simulink model "BLDC_Completo"  (R2024b)
settings: Solver=ode23s  StartTime=0.0  StopTime=3  MaxStep=1e-4  RelTol=1e-3
values from neighbouring files (symbols this model uses):
  b_eq = b_l*(1/r)^2+b_m    (= 2.36823386114e-05)    [Parametros.m]
  c_pitch = cos(pitch)    [Parametros.m]
  J_eq = J_l*(1/r)^2+J_m    (= 7.12145792242e-06)    [Parametros.m]
  K_e = 0.0217    [Parametros.m]
  k_l = m*g*l_cm+m_l*g*l_l    (= 5.05042475)    [Parametros.m]
  K_t = 21.7e-3    (= 0.0217)    [Parametros.m]
  Kd_m = J_eq*n*w_pos    (= 0.0159520657462)    [Parametros.m]
  ke_int = w_obs^3    (= 125000000000)    [Parametros.m]
  ke_tita = w_obs*3    (= 15000)    [Parametros.m]
  ke_w = 3*w_obs^2    (= 75000000)    [Parametros.m]
  Ki_m = J_eq*w_pos^3    (= 3646.18645628)    [Parametros.m]
  Kp_m = J_eq*n*w_pos^2    (= 12.761652597)    [Parametros.m]
  L_s = 0.113e-3    (= 0.000113)    [Parametros.m]
  p = 7    [Parametros.m]
  p_i = -5000    [Parametros.m]
  psi_m = K_e/(1.5*p)    (= 0.00206666666667)    [Parametros.m]
  r = 156    [Parametros.m]
  R_s = 0.196    [Parametros.m]
  s_pitch = sin(pitch)    [Parametros.m]
  s_roll = sin(roll)    [Parametros.m]
settings Model: Creator=ribei  LastModifiedBy=ribei
settings DataIOCC: ExternalInput=q_vel  LoadExternalInput=on

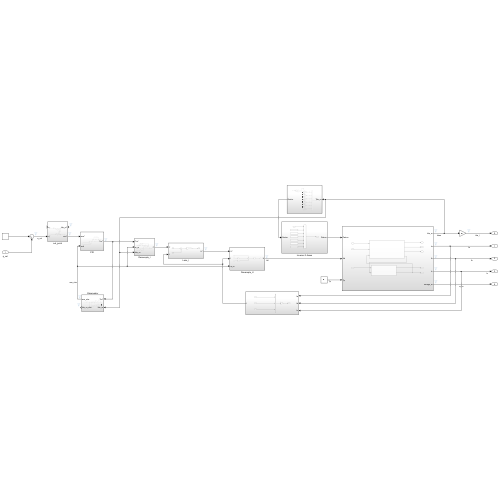
[thumbnail: Simulink's stored preview of the top-level diagram]
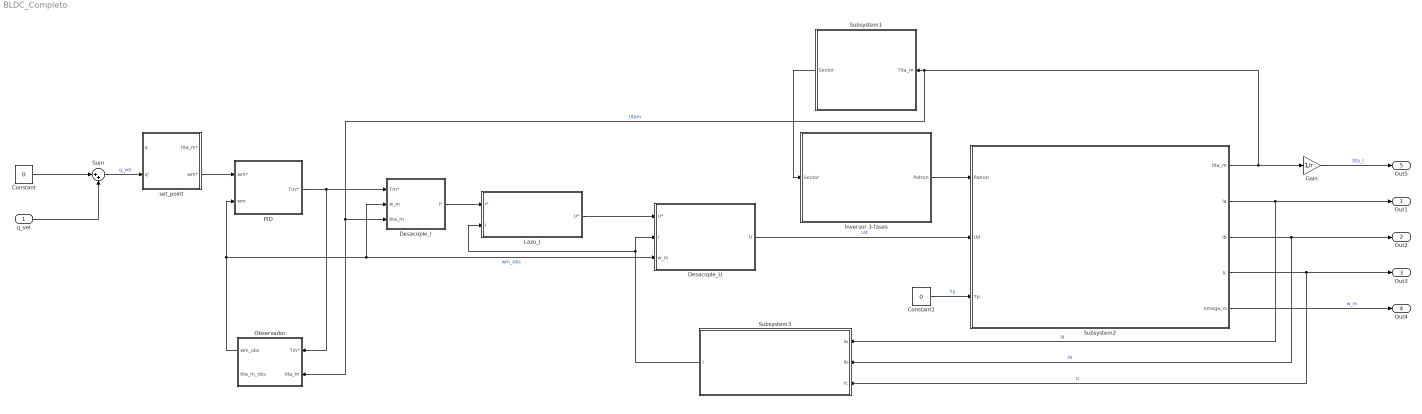
== system BLDC_Completo ==
  q_vel : Inport
  Constant : Constant  Value=0
  Constant1 : Constant  Value=0
  Desacople_I : Subsystem
  Desacople_U : Subsystem
  Gain : Gain  Gain=1/r
  Inversor 3-fases : Subsystem
  Lazo_I : Subsystem
  Observador : Subsystem
  PID : Subsystem
  Subsystem1 : Subsystem
  Subsystem2 : Subsystem
  Subsystem3 : Subsystem
  Sum : Sum  Inputs=|++
  set_point : Subsystem
  Out1 : Outport
  Out2 : Outport  Port=2
  Out3 : Outport  Port=3
  Out4 : Outport  Port=4
  Out5 : Outport  Port=5
  wires:
  Subsystem2/4(Ic) -> Subsystem3/3(Ic), Out3/1  "Ic"
  Lazo_I/1(U*) -> Desacople_U/1(U*)
  set_point/2(wm*) -> PID/1(wm*)
  Sum/1 -> set_point/2(q')  "q_vel"
  Subsystem2/5(omega_m) -> Out4/1  "w_m"
  Subsystem1/1(Sector) -> Inversor 3-fases/1(Sector)
  Subsystem3/1(I) -> Lazo_I/2(I), Desacople_U/2(I)
  Desacople_U/1(U) -> Subsystem2/2(Ud)  "Ud"
  Subsystem2/3(Ib) -> Subsystem3/2(Ib), Out2/1  "Ib"
  Subsystem2/1(tita_m) -> Observador/2(tita_m), Desacople_I/3(tita_m), Subsystem1/1(Tita_m), Gain/1  "titam"
  Constant1/1 -> Subsystem2/3(Tp)  "Tp"
  Subsystem2/2(Ia) -> Subsystem3/1(Ia), Out1/1  "Ia"
  PID/1(Tm*') -> Desacople_I/1(Tm*), Observador/1(Tm*)
  Inversor 3-fases/1(Patron) -> Subsystem2/1(Patron)
  q_vel/1 -> Sum/2
  Desacople_I/1(I*) -> Lazo_I/1(I*)
  Observador/1(wm_obs) -> Desacople_I/2(w_m), Desacople_U/3(w_m), PID/2(wm)  "wm_obs"
  Constant/1 -> Sum/1
  Gain/1 -> Out5/1  "tita_l"

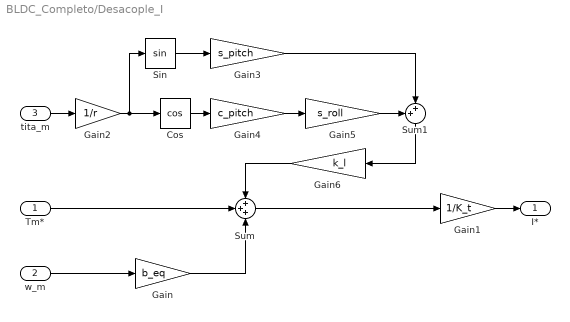
== system BLDC_Completo/Desacople_I ==
  Tm* : Inport
  w_m : Inport  Port=2
  tita_m : Inport  Port=3
  Cos : Trigonometry  Operator=cos
  Gain : Gain  Gain=b_eq
  Gain1 : Gain  Gain=1/K_t
  Gain2 : Gain  Gain=1/r
  Gain3 : Gain  Gain=s_pitch
  Gain4 : Gain  Gain=c_pitch
  Gain5 : Gain  Gain=s_roll
  Gain6 : Gain  Gain=k_l
  Sin : Trigonometry
  Sum : Sum  Inputs=+++
  Sum1 : Sum  Inputs=++|
  I* : Outport
  wires:
  w_m/1 -> Gain/1
  Gain/1 -> Sum/3
  Sum/1 -> Gain1/1
  Gain1/1 -> I*/1
  Gain2/1 -> Cos/1, Sin/1
  tita_m/1 -> Gain2/1
  Cos/1 -> Gain4/1
  Sin/1 -> Gain3/1
  Sum1/1 -> Gain6/1
  Gain4/1 -> Gain5/1
  Gain5/1 -> Sum1/1
  Gain3/1 -> Sum1/2
  Gain6/1 -> Sum/1
  Tm*/1 -> Sum/2

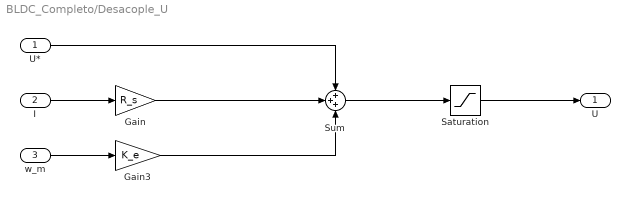
== system BLDC_Completo/Desacople_U ==
  U* : Inport
  I : Inport  Port=2
  w_m : Inport  Port=3
  Gain : Gain  Gain=R_s
  Gain3 : Gain  Gain=K_e
  Saturation : Saturate  UpperLimit=18  LowerLimit=-18
  Sum : Sum  Inputs=+++
  U : Outport
  wires:
  I/1 -> Gain/1
  w_m/1 -> Gain3/1
  Gain/1 -> Sum/2
  U*/1 -> Sum/1
  Gain3/1 -> Sum/3
  Sum/1 -> Saturation/1
  Saturation/1 -> U/1

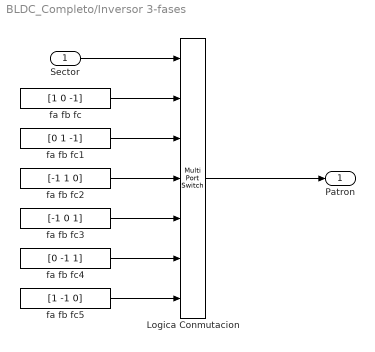
== system BLDC_Completo/Inversor 3-fases ==
  Sector : Inport
  Logica Conmutacion : MultiPortSwitch  Inputs=6  DiagnosticForDefault=None  SaturateOnIntegerOverflow=off  InputSameDT=off
  fa fb fc : Constant  Value=[1 0 -1]
  fa fb fc1 : Constant  Value=[0 1 -1]
  fa fb fc2 : Constant  Value=[-1 1 0]
  fa fb fc3 : Constant  Value=[-1 0 1]
  fa fb fc4 : Constant  Value=[0 -1 1]
  fa fb fc5 : Constant  Value=[1 -1 0]
  Patron : Outport
  wires:
  Logica Conmutacion/1 -> Patron/1
  fa fb fc2/1 -> Logica Conmutacion/4
  fa fb fc5/1 -> Logica Conmutacion/7
  Sector/1 -> Logica Conmutacion/1
  fa fb fc3/1 -> Logica Conmutacion/5
  fa fb fc4/1 -> Logica Conmutacion/6
  fa fb fc1/1 -> Logica Conmutacion/3
  fa fb fc/1 -> Logica Conmutacion/2

== system BLDC_Completo/Lazo_I ==
  I* : Inport
  I : Inport  Port=2
  Gain : Gain  Gain=-p_i*L_s
  Sum : Sum  Inputs=|+-
  U* : Outport
  wires:
  I*/1 -> Sum/1
  I/1 -> Sum/2
  Gain/1 -> U*/1
  Sum/1 -> Gain/1

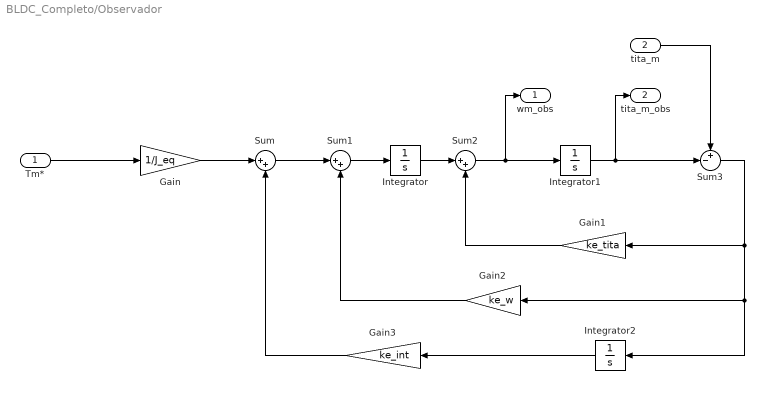
== system BLDC_Completo/Observador ==
  Tm* : Inport
  tita_m : Inport  Port=2
  Gain : Gain  Gain=1/J_eq
  Gain1 : Gain  Gain=ke_tita
  Gain2 : Gain  Gain=ke_w
  Gain3 : Gain  Gain=ke_int
  Integrator : Integrator
  Integrator1 : Integrator  InitialCondition=pi/6
  Integrator2 : Integrator
  Sum : Sum  Inputs=|++
  Sum1 : Sum  Inputs=|++
  Sum2 : Sum  Inputs=|++
  Sum3 : Sum  Inputs=+-|
  wm_obs : Outport
  tita_m_obs : Outport  Port=2
  wires:
  Tm*/1 -> Gain/1
  Gain/1 -> Sum/1
  Sum/1 -> Sum1/1
  Sum1/1 -> Integrator/1
  Integrator/1 -> Sum2/1
  Sum2/1 -> wm_obs/1, Integrator1/1
  Integrator1/1 -> tita_m_obs/1, Sum3/2
  tita_m/1 -> Sum3/1
  Sum3/1 -> Gain1/1, Gain2/1, Integrator2/1
  Gain1/1 -> Sum2/2
  Gain2/1 -> Sum1/2
  Integrator2/1 -> Gain3/1
  Gain3/1 -> Sum/2

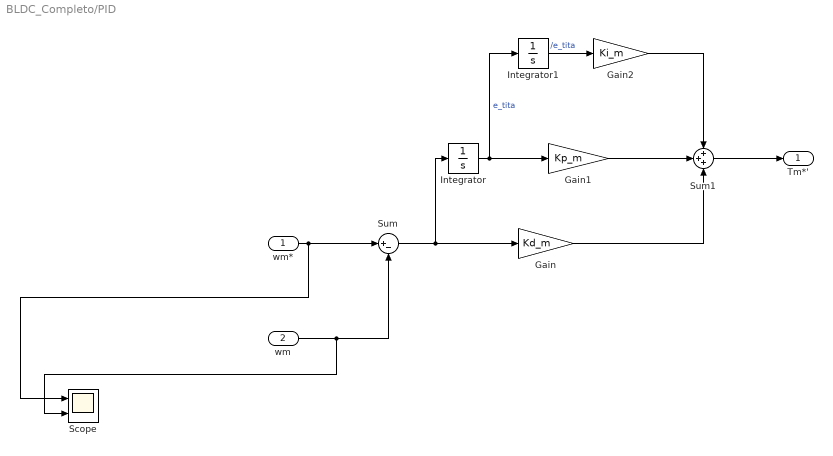
== system BLDC_Completo/PID ==
  wm* : Inport
  wm : Inport  Port=2
  Gain : Gain  Gain=Kd_m
  Gain1 : Gain  Gain=Kp_m
  Gain2 : Gain  Gain=Ki_m
  Integrator : Integrator
  Integrator1 : Integrator
  Scope : Scope  NumInputPorts=2
  Sum : Sum  Inputs=|+-
  Sum1 : Sum  Inputs=+++
  Tm*' : Outport
  wires:
  Gain2/1 -> Sum1/1
  Gain/1 -> Sum1/3
  Gain1/1 -> Sum1/2
  Sum1/1 -> Tm*'/1
  wm/1 -> Scope/2, Sum/2
  Integrator/1 -> Gain1/1, Integrator1/1  "e_tita"
  Integrator1/1 -> Gain2/1  "/e_tita"
  wm*/1 -> Scope/1, Sum/1
  Sum/1 -> Gain/1, Integrator/1

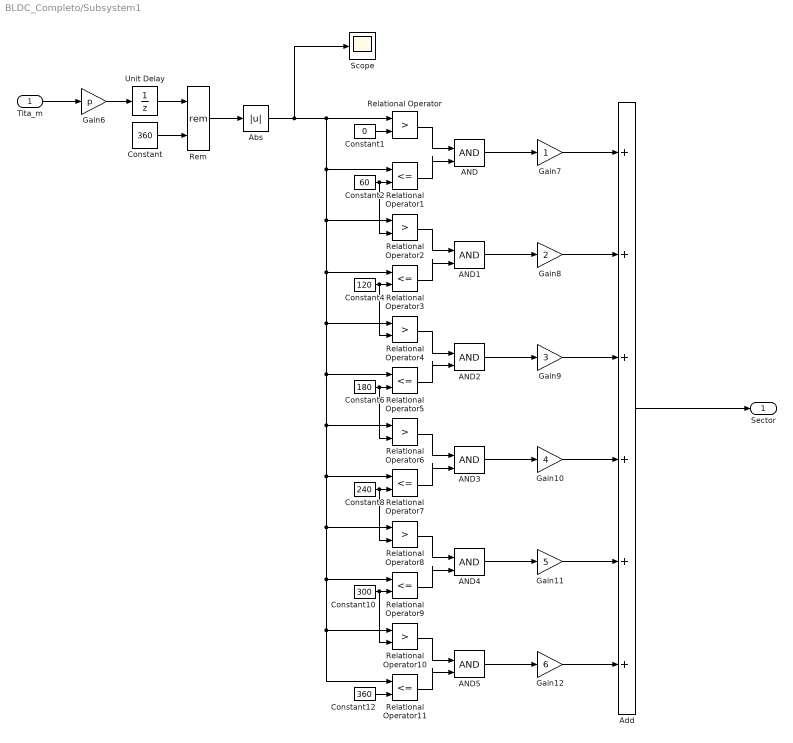
== system BLDC_Completo/Subsystem1 ==
  Tita_m : Inport
  AND{,1..5} (6 alike) : Logic  IconShape=distinctive  AllPortsSameDT=off  OutDataTypeStr=boolean
  Abs : Abs  SaturateOnIntegerOverflow=off
  Add : Sum  Inputs=++++++
  Constant : Constant  Value=360
  Constant1 : Constant  Value=0
  Constant10 : Constant  Value=300
  Constant12 : Constant  Value=360
  Constant2 : Constant  Value=60
  Constant4 : Constant  Value=120
  Constant6 : Constant  Value=180
  Constant8 : Constant  Value=240
  Gain10 : Gain  Gain=4
  Gain11 : Gain  Gain=5
  Gain12 : Gain  Gain=6
  Gain6 : Gain  Gain=p
  Gain7 : Gain
  Gain8 : Gain  Gain=2
  Gain9 : Gain  Gain=3
  Relational Operator{,2,4,6,8,10} (6 alike) : RelationalOperator  Operator=>  OutDataTypeStr=boolean  RndMeth=Simplest  InputSameDT=off
  Relational Operator{1,3,5,7,9,11} (6 alike) : RelationalOperator  Operator=<=  OutDataTypeStr=boolean  RndMeth=Simplest  InputSameDT=off
  Rem : Math  Operator=rem
  Scope : Scope
  Unit Delay : UnitDelay  SampleTime=0.001  HasFrameUpgradeWarning=on
  Sector : Outport
  wires:
  Rem/1 -> Abs/1
  AND4/1 -> Gain11/1
  AND1/1 -> Gain8/1
  Relational Operator4/1 -> AND2/1
  Add/1 -> Sector/1
  Gain10/1 -> Add/4
  Relational Operator8/1 -> AND4/1
  Relational Operator3/1 -> AND1/2
  Relational Operator2/1 -> AND1/1
  Gain9/1 -> Add/3
  Constant4/1 -> Relational Operator4/2, Relational Operator3/2
  Constant6/1 -> Relational Operator6/2, Relational Operator5/2
  Gain11/1 -> Add/5
  Constant2/1 -> Relational Operator2/2, Relational Operator1/2
  AND2/1 -> Gain9/1
  Gain7/1 -> Add/1
  Relational Operator5/1 -> AND2/2
  Constant10/1 -> Relational Operator10/2, Relational Operator9/2
  AND/1 -> Gain7/1
  Constant1/1 -> Relational Operator/2
  Relational Operator/1 -> AND/1
  Constant/1 -> Rem/2
  Relational Operator11/1 -> AND5/2
  Constant12/1 -> Relational Operator11/2
  Relational Operator10/1 -> AND5/1
  AND5/1 -> Gain12/1
  Relational Operator9/1 -> AND4/2
  Unit Delay/1 -> Rem/1
  Gain12/1 -> Add/6
  Gain6/1 -> Unit Delay/1
  Tita_m/1 -> Gain6/1
  Constant8/1 -> Relational Operator8/2, Relational Operator7/2
  Relational Operator1/1 -> AND/2
  Relational Operator7/1 -> AND3/2
  AND3/1 -> Gain10/1
  Relational Operator6/1 -> AND3/1
  Gain8/1 -> Add/2
  Abs/1 -> Scope/1, Relational Operator/1, Relational Operator1/1, Relational Operator2/1, Relational Operator3/1, Relational Operator4/1, Relational Operator5/1, Relational Operator6/1, Relational Operator7/1, Relational Operator8/1, Relational Operator9/1, Relational Operator10/1, Relational Operator11/1

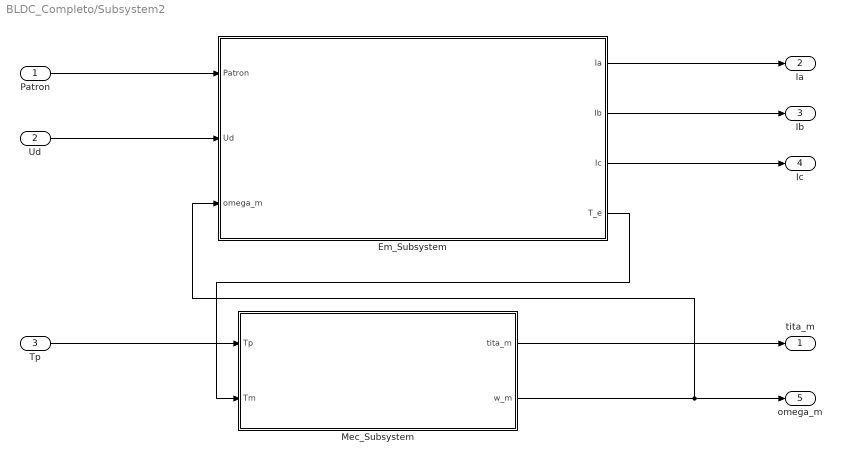
== system BLDC_Completo/Subsystem2 ==
  Patron : Inport
  Ud : Inport  Port=2
  Tp : Inport  Port=3
  Em_Subsystem : Subsystem
  Mec_Subsystem : Subsystem
  tita_m : Outport
  Ia : Outport  Port=2
  Ib : Outport  Port=3
  Ic : Outport  Port=4
  omega_m : Outport  Port=5
  wires:
  Mec_Subsystem/1(tita_m) -> tita_m/1
  Patron/1 -> Em_Subsystem/1(Patron)
  Mec_Subsystem/2(w_m) -> omega_m/1, Em_Subsystem/3(omega_m)
  Em_Subsystem/4(T_e) -> Mec_Subsystem/2(Tm)
  Tp/1 -> Mec_Subsystem/1(Tp)
  Em_Subsystem/1(Ia) -> Ia/1
  Em_Subsystem/3(Ic) -> Ic/1
  Em_Subsystem/2(Ib) -> Ib/1
  Ud/1 -> Em_Subsystem/2(Ud)

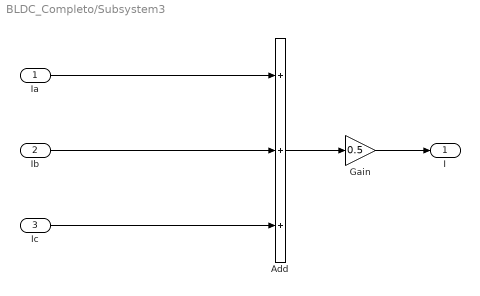
== system BLDC_Completo/Subsystem3 ==
  Ia : Inport
  Ib : Inport  Port=2
  Ic : Inport  Port=3
  Add : Sum  Inputs=+++
  Gain : Gain  Gain=0.5
  I : Outport
  wires:
  Ia/1 -> Add/1
  Ic/1 -> Add/3
  Ib/1 -> Add/2
  Add/1 -> Gain/1
  Gain/1 -> I/1

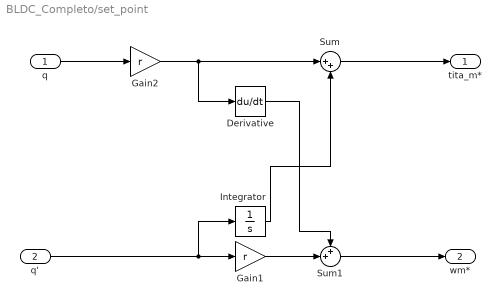
== system BLDC_Completo/set_point ==
  q : Inport
  q' : Inport  Port=2
  Derivative : Derivative
  Gain1 : Gain  Gain=r
  Gain2 : Gain  Gain=r
  Integrator : Integrator
  Sum : Sum  Inputs=|++
  Sum1 : Sum  Inputs=++|
  tita_m* : Outport
  wm* : Outport  Port=2
  wires:
  Gain2/1 -> Derivative/1, Sum/1
  Sum/1 -> tita_m*/1
  q/1 -> Gain2/1
  Derivative/1 -> Sum1/1
  q'/1 -> Integrator/1, Gain1/1
  Sum1/1 -> wm*/1
  Integrator/1 -> Sum/2
  Gain1/1 -> Sum1/2

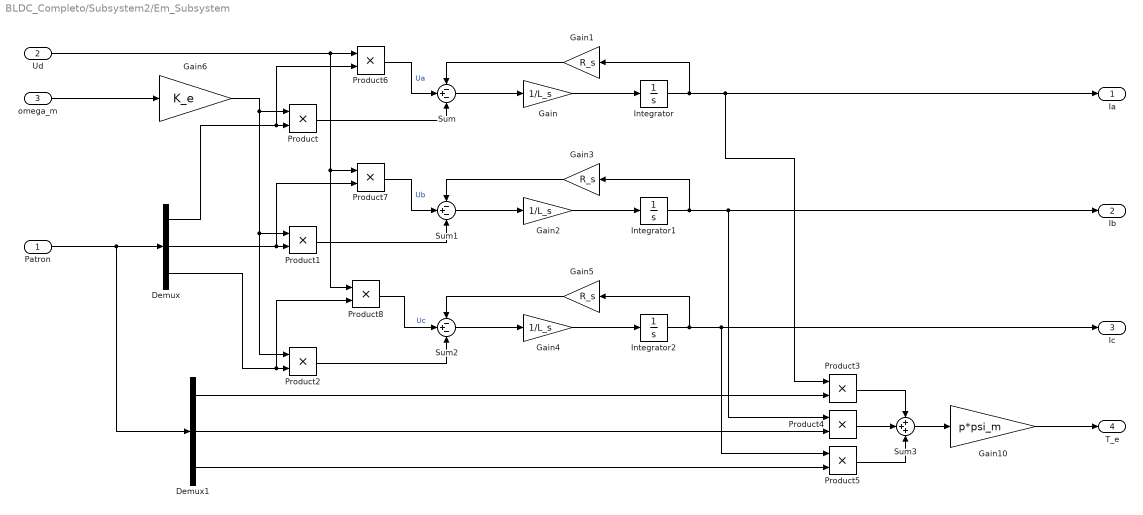
== system BLDC_Completo/Subsystem2/Em_Subsystem ==
  Patron : Inport
  Ud : Inport  Port=2
  omega_m : Inport  Port=3
  Demux : Demux  Outputs=3
  Demux1 : Demux  Outputs=3
  Gain : Gain  Gain=1/L_s
  Gain1 : Gain  Gain=R_s
  Gain10 : Gain  Gain=p*psi_m
  Gain2 : Gain  Gain=1/L_s
  Gain3 : Gain  Gain=R_s
  Gain4 : Gain  Gain=1/L_s
  Gain5 : Gain  Gain=R_s
  Gain6 : Gain  Gain=K_e
  Integrator : Integrator
  Integrator1 : Integrator
  Integrator2 : Integrator
  Product{,1..8} (9 alike) : Product
  Sum : Sum  Inputs=-+-
  Sum1 : Sum  Inputs=-+-
  Sum2 : Sum  Inputs=-+-
  Sum3 : Sum  Inputs=+++
  Ia : Outport
  Ib : Outport  Port=2
  Ic : Outport  Port=3
  T_e : Outport  Port=4
  wires:
  Gain/1 -> Integrator/1
  Integrator/1 -> Gain1/1, Product3/1, Ia/1
  Sum/1 -> Gain/1
  Gain1/1 -> Sum/1
  Sum1/1 -> Gain2/1
  Gain3/1 -> Sum1/1
  Gain2/1 -> Integrator1/1
  Integrator1/1 -> Product4/1, Ib/1, Gain3/1
  Gain4/1 -> Integrator2/1
  Gain5/1 -> Sum2/1
  Sum2/1 -> Gain4/1
  Integrator2/1 -> Product5/1, Ic/1, Gain5/1
  omega_m/1 -> Gain6/1
  Gain6/1 -> Product/1, Product1/1, Product2/1
  Demux/1 -> Product6/2, Product/2
  Demux/2 -> Product7/2, Product1/2
  Demux/3 -> Product8/2, Product2/2
  Product/1 -> Sum/3
  Product1/1 -> Sum1/3
  Product2/1 -> Sum2/3
  Patron/1 -> Demux1/1, Demux/1
  Demux1/1 -> Product3/2
  Demux1/2 -> Product4/2
  Demux1/3 -> Product5/2
  Product3/1 -> Sum3/1
  Product4/1 -> Sum3/2
  Product5/1 -> Sum3/3
  Sum3/1 -> Gain10/1
  Gain10/1 -> T_e/1
  Ud/1 -> Product8/1, Product7/1, Product6/1
  Product6/1 -> Sum/2  "Ua"
  Product7/1 -> Sum1/2  "Ub"
  Product8/1 -> Sum2/2  "Uc"

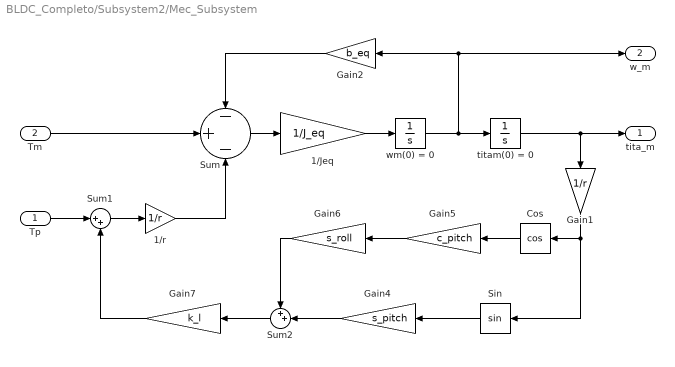
== system BLDC_Completo/Subsystem2/Mec_Subsystem ==
  Tp : Inport
  Tm : Inport  Port=2
  1/Jeq : Gain  Gain=1/J_eq
  1/r : Gain  Gain=1/r
  Cos : Trigonometry  Operator=cos
  Gain1 : Gain  Gain=1/r
  Gain2 : Gain  Gain=b_eq
  Gain4 : Gain  Gain=s_pitch
  Gain5 : Gain  Gain=c_pitch
  Gain6 : Gain  Gain=s_roll
  Gain7 : Gain  Gain=k_l
  Sin : Trigonometry
  Sum : Sum  Inputs=-+-
  Sum1 : Sum  Inputs=|++
  Sum2 : Sum  Inputs=++|
  titam(0) = 0 : Integrator  InitialCondition=pi/6
  wm(0) = 0 : Integrator
  tita_m : Outport
  w_m : Outport  Port=2
  wires:
  wm(0) = 0/1 -> Gain2/1, w_m/1, titam(0) = 0/1
  1/r/1 -> Sum/3
  titam(0) = 0/1 -> Gain1/1, tita_m/1
  Tp/1 -> Sum1/1
  Sum1/1 -> 1/r/1
  Tm/1 -> Sum/2
  Gain2/1 -> Sum/1
  Sum/1 -> 1/Jeq/1
  1/Jeq/1 -> wm(0) = 0/1
  Cos/1 -> Gain5/1
  Gain4/1 -> Sum2/2
  Gain6/1 -> Sum2/1
  Sin/1 -> Gain4/1
  Gain5/1 -> Gain6/1
  Gain1/1 -> Cos/1, Sin/1
  Sum2/1 -> Gain7/1
  Gain7/1 -> Sum1/2
